simulink model "sldemo_bounce"  (R2023b)
settings: Solver=ode23  StartTime=0.0  StopTime=25  MaxStep=0.01  RelTol=1e-3  AbsTol=1E-6  EnableMultiTasking=on
PreLoadFcn:
  | k = -0.8;
Description:
  | Bouncing Ball Model
  | 
  | This model calculates the trajectory, over time, of a ball thrown
  | upward with a velocity of 15 meters per second from a height of 10 m.
  | The model demonstrates the use of the 'ReinitDXDTwhenXreachesSaturation'
  | parameter in the Second-Order Integrator block to model this system.
  | This parameter, when set to 'on', forces a reinitialization of dx/dt
  | (velocity in the model) at the instant when x (position) reaches
  | saturation (i.e., when the ball hits the ground). The reinitialized value
  | is calculated by multiplying a coefficient of restitution times the ball
  | velocity, the instant before the ball hits the ground. The Memory block
  | in the calculation loop serves to capture the velocity of the ball just
  | before it hits the ground. The position of the ball is plotted in the
  | upper axis of the scope while the velocity of the ball is plotted in
  | the lower axis.
settings Model: ModifiedByFormat=The MathWorks, Inc.  Creator=The MathWorks, Inc.  LastModifiedBy=The MathWorks, Inc.
settings SolverCC: AutoScaleAbsTol=off  AlgebraicLoopSolver=TrustRegion
settings DataIOCC: MaxDataPoints=7500  SaveFormat=Array  SaveOutput=off  DSMLogging=off  SaveTime=off  ReturnWorkspaceOutputs=off
settings OptimizationCC: ReuseModelBlockBuffer=off  ExpressionDepthLimit=2147483647  EfficientFloat2IntCast=on  LifeSpan=inf
settings DebuggingCC: UnderspecifiedInitializationDetection=Classic  MergeDetectMultiDrivingBlocksExec=none  IgnoredZcDiagnostic=none  FcnCallInpInsideContextMsg=warning  UnconnectedInputMsg=warning  UnconnectedOutputMsg=warning  UnconnectedLineMsg=warning  StateNameClashWarn=warning  SFUnexpectedBacktrackingDiag=warning  SFNoUnconditionalDefaultTransitionDiag=warning  SFExecutionAtInitializationDiag=none  ArithmeticOperatorsInVariantConditions=warning
settings HardwareCC: ProdBitPerPointer=32  ProdBitPerSizeT=32  ProdBitPerPtrDiffT=32  ProdLargestAtomicFloat=None  ProdIntDivRoundTo=Undefined  ProdEndianess=Unspecified  ProdWordSize=32  ProdHWDeviceType=32-bit Generic  TargetBitPerPointer=64  TargetBitPerSizeT=64  TargetBitPerPtrDiffT=64  TargetLongLongMode=on  TargetIntDivRoundTo=Zero  TargetEndianess=LittleEndian  TargetWordSize=64  TargetHWDeviceType=MATLAB Host  ProdEqTarget=off
settings ModelReferenceCC: EnableRefExpFcnMdlSchedulingChecks=on  PropagateSignalLabelsOutOfModel=off
settings SFSimCC: SimUseLocalCustomCode=off  CustomCodeUndefinedFunction=UseInterfaceOnly
settings RTWCC: Description=Rapid Simulation Target  SystemTargetFile=rsim.tlc  TemplateMakefile=rsim_default_tmf  RTWUseLocalCustomCode=off
settings CodeAppCC: StateflowObjectComments=on
settings RSimTargetCC: OptimizeReductions=off
settings ConfigComp: CovMetricSettings=dw  CovSaveCumulativeToWorkspaceVar=on  CovSaveSingleToWorkspaceVar=on  CovExternalEMLEnable=off

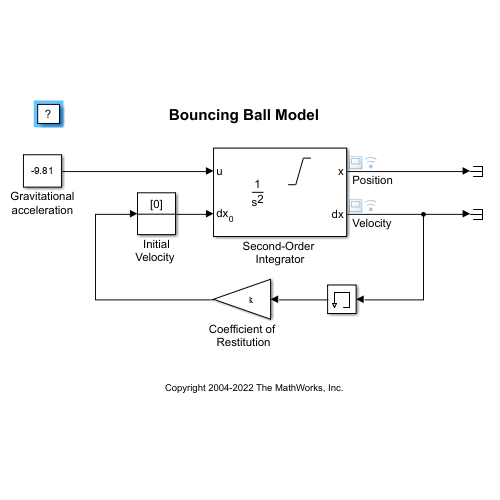
[thumbnail: Simulink's stored preview of the top-level diagram]
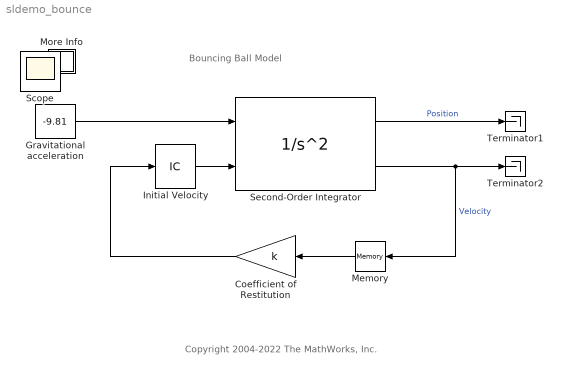
== system sldemo_bounce ==
  note: Bouncing Ball Model
  note: Copyright 2004-2022 The MathWorks, Inc.
  Coefficient of Restitution : Gain  Gain=k
  Gravitational acceleration : Constant  Value=-9.81  OutDataTypeStr=double
  "Initial Velocity " : InitialCondition  Value=0
  Memory : Memory
  More Info : Subsystem
      settings: OpenFcn=showExample('simulink_general/sldemo_bounceExample')
      mask Display: disp('?')
  Second-Order Integrator : SecondOrderIntegrator  ICX=25.0  LimitX=on  LowerLimitX=0.0  StateNameX='Position'  ICSourceDXDT=external  StateNameDXDT='Velocity'  ReinitDXDTwhenXreachesSaturation=on
  Terminator1 : Terminator
  Terminator2 : Terminator
  Scope : Scope
  wires:
  Gravitational acceleration/1 -> Second-Order Integrator/1
  Second-Order Integrator/1 -> Terminator1/1  "Position"
  Second-Order Integrator/2 -> Memory/1, Terminator2/1  "Velocity"
  Memory/1 -> Coefficient of Restitution/1
  "Initial Velocity "/1 -> Second-Order Integrator/2
  Coefficient of Restitution/1 -> "Initial Velocity "/1

== system sldemo_bounce/More Info ==
